simulink model "project_ElectricMotor"  (R2019a)
settings: Solver=FixedStepAuto  StartTime=0.0  StopTime=10.0  FixedStep=0.001  RelTol=1e-3
undefined symbols (not defined in the file): B, KePhi, Ra, T_a, T_L, T_m, Va
libraries: simulink_extras x2
settings Model: Creator=ansar  LastModifiedBy=ansar

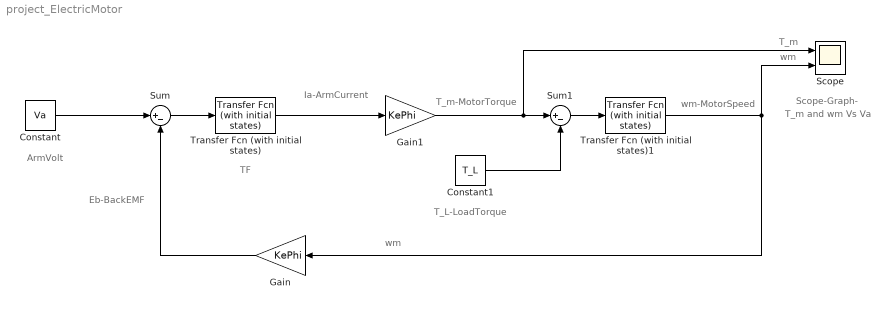
== system project_ElectricMotor ==
  note: wm
  note: T_m
  note: T_m and wm Vs Va
  note: Scope-Graph-
  note: T_m-MotorTorque
  note: T_L-LoadTorque
  note: wm-MotorSpeed
  note: TF
  note: Eb-BackEMF
  note: wm
  note: ArmVolt
  note: Ia-ArmCurrent
  Constant : Constant  Value=Va
  Constant1 : Constant  Value=T_L
  Gain : Gain  Gain=KePhi
  Gain1 : Gain  Gain=KePhi
  Scope : Scope  NumInputPorts=2
  Sum : Sum  Inputs=|+-
  Sum1 : Sum  Inputs=|+-
  Transfer Fcn (with initial states) : simulink_extras/Additional Linear/Transfer Fcn (with initial states)  N=[1/Ra]  D="[T_a  1]"  X0=.5
  Transfer Fcn (with initial states)1 : simulink_extras/Additional Linear/Transfer Fcn (with initial states)  N=[1/B]  D="[T_m  1]"  X0=.5
  wires:
  Constant/1 -> Sum/1
  Gain/1 -> Sum/2
  Transfer Fcn (with initial states)1/1 -> Scope/2, Gain/1
  Sum/1 -> Transfer Fcn (with initial states)/1
  Transfer Fcn (with initial states)/1 -> Gain1/1
  Gain1/1 -> Sum1/1, Scope/1
  Constant1/1 -> Sum1/2
  Sum1/1 -> Transfer Fcn (with initial states)1/1
